simulink model "nonlinear_simulation"  (R2020b)
settings: Solver=ode23t  StartTime=0.0  StopTime=30  MaxStep=0.01  RelTol=1e-7
StopFcn:
  | run plot_simulation_results
values from neighbouring files (symbols this model uses):
  G_hov = [ 0 0 0 0 0 0 1 0 ]    [compute_linear_controller.m]
  G_pos = [ 1 0 0 0 ... (first row only)    [compute_linear_controller.m]
  int_lim = wt/K_hov(5,9) + wt*0.005    [compute_linear_controller.m]
  K_hov = lqr(sys_int, Q, R)    [compute_linear_controller.m]
  K_pos = lqr(sys_hint, Q_pos, R_pos)    [compute_linear_controller.m]
libraries: simulink x1
settings Model: Creator=theso  LastModifiedBy=Emil

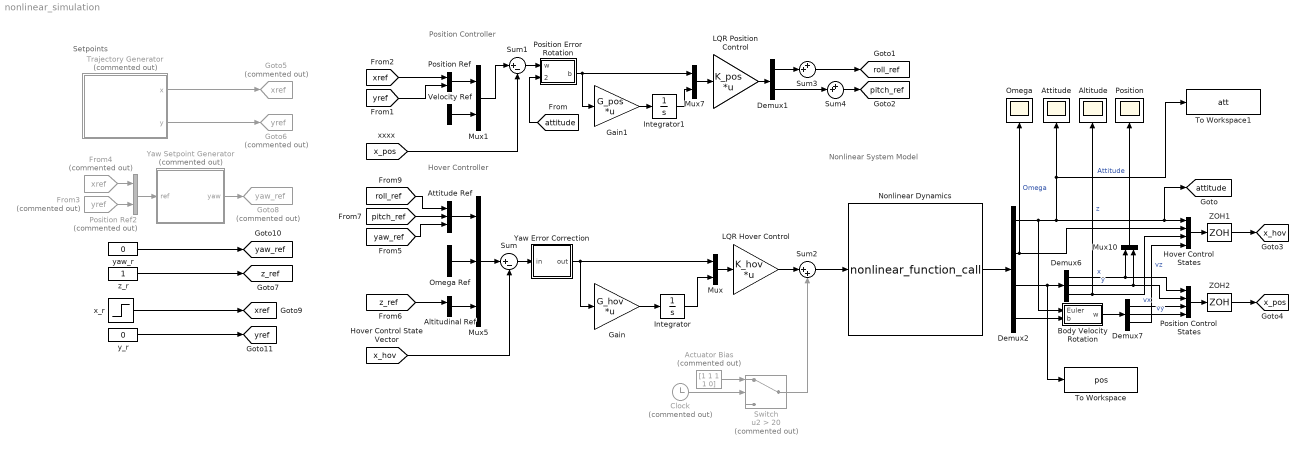
== system nonlinear_simulation ==
  note: Position Controller
  note: Nonlinear System Model
  note: Hover Controller
  note: Setpoints
  Actuator Bias : Constant  Commented=on  Value=[1 1 1 1 0]
  Altitude : Scope
  Altitudinal Ref : Mux  Inputs=2
  Attitude : Scope
  Attitude Ref : Mux  Inputs=3
  Body Velocity Rotation : Subsystem
  Clock : Clock  Commented=on
  Demux1 : Demux  Outputs=2
  Demux2 : Demux
  Demux6 : Demux  Outputs=3
  Demux7 : Demux  Outputs=3
  From3 : From  Commented=on  GotoTag=yref  TagVisibility=global
  From4 : From  Commented=on  GotoTag=xref  TagVisibility=global
  Gain : Gain  Gain=G_hov  Multiplication=Matrix(K*u)
  Gain1 : Gain  Gain=G_pos  Multiplication=Matrix(K*u)
  Goto5 : Goto  Commented=on  GotoTag=xref  TagVisibility=global
  Goto6 : Goto  Commented=on  GotoTag=yref  TagVisibility=global
  Goto8 : Goto  Commented=on  GotoTag=yaw_ref  TagVisibility=global
  Hover Control States : Mux
  Integrator : Integrator  LimitOutput=on  UpperSaturationLimit=int_lim  LowerSaturationLimit=0
  Integrator1 : Integrator  LimitOutput=on  UpperSaturationLimit=0.4  LowerSaturationLimit=-0.4
  LQR Hover Control : Gain  Gain=K_hov  Multiplication=Matrix(K*u)
  LQR Position Control : Gain  Gain=K_pos  Multiplication=Matrix(K*u)
  Mux{,1,7,10} (4 alike) : Mux  Inputs=2
  Mux5 : Mux  Inputs=3
  Nonlinear Dynamics : S-Function  FunctionName=nonlinear_function_call  SFunctionDeploymentMode=off  EnableBusSupport=off
      mask Display: image('drone_model_icon.png'); % Use "Edit Image" on toolstrip to change.
  Omega : Scope
  Omega Ref : Mux  Inputs=3
  Position : Scope
  Position Control States : Mux
  Position Error Rotation : Subsystem
  Position Ref : Mux  Inputs=2
  Position Ref2 : Mux  Commented=on  Inputs=2
  Sum : Sum  Inputs=|+-
  Sum1 : Sum  Inputs=|+-
  Sum2 : Sum  Inputs=|++
  Sum3 : Sum  Inputs=++|
  Sum4 : Sum  Inputs=++|
  Switch : Switch  Commented=on  Criteria=u2 > Threshold  Threshold=20
  To Workspace : ToWorkspace  VariableName=pos  SaveFormat=Timeseries  SampleTime=-1
  To Workspace1 : ToWorkspace  VariableName=att  SaveFormat=Timeseries  SampleTime=-1
  Trajectory Generator : Subsystem  Commented=on
  Velocity Ref : Mux  Inputs=2
  Yaw Error Correction : Subsystem
  Yaw Setpoint Generator : MATLAB Function  Commented=on  TreatAsAtomicUnit=on
  ZOH1 : ZeroOrderHold  SampleTime=0.005
  ZOH2 : ZeroOrderHold  SampleTime=0.005
  x_r : Step  Time=10  SampleTime=0
  y_r : Constant  Value=0
  yaw_r : Constant  Value=0
  z_r : Constant
  tag scope: attitude=global, pitch_ref=global, roll_ref=global, x_hov=global, x_pos=global, xref=global, yaw_ref=global, yref=global, z_ref=global
  wires:
  Mux5/1 -> Sum/1
  Sum/1 -> Yaw Error Correction/1(in)
  Gain/1 -> Integrator/1
  Mux/1 -> LQR Hover Control/1
  Integrator/1 -> Mux/2
  Mux1/1 -> Sum1/1
  Mux7/1 -> LQR Position Control/1
  Nonlinear Dynamics/1 -> Demux2/1
  Demux2/1 -> To Workspace1/1, Attitude/1, [attitude], Hover Control States/1, Body Velocity Rotation/1(Euler)  "Attitude"
  Demux2/2 -> Hover Control States/2, Omega/1  "Omega"
  Demux2/4 -> Body Velocity Rotation/2(b)
  Body Velocity Rotation/1(w) -> Demux7/1
  Demux7/1 -> Position Control States/3  "vx"
  Demux7/2 -> Position Control States/4  "vy"
  Demux6/1 -> Position Control States/1, Mux10/1  "x"
  Demux6/2 -> Mux10/2, Position Control States/2  "y"
  Demux7/3 -> Hover Control States/4  "vz"
  Demux6/3 -> Hover Control States/3, Altitude/1  "z"
  Mux10/1 -> Position/1
  Attitude Ref/1 -> Mux5/1
  Omega Ref/1 -> Mux5/2
  Altitudinal Ref/1 -> Mux5/3
  Velocity Ref/1 -> Mux1/2
  LQR Position Control/1 -> Demux1/1
  Gain1/1 -> Integrator1/1
  Integrator1/1 -> Mux7/2
  Position Ref/1 -> Mux1/1
  Sum1/1 -> Position Error Rotation/1(w)
  Position Error Rotation/1(b) -> Mux7/1, Gain1/1
  Yaw Error Correction/1(out) -> Gain/1, Mux/1
  Demux2/3 -> To Workspace/1, Demux6/1
  [z_ref] -> Altitudinal Ref/1
  [xref] -> Position Ref/1
  [yref] -> Position Ref/2
  [attitude] -> Position Error Rotation/2(Euler)
  From3/1 -> Position Ref2/2
  From4/1 -> Position Ref2/1
  Position Ref2/1 -> Yaw Setpoint Generator/1(ref)
  [yaw_ref] -> Attitude Ref/3
  [roll_ref] -> Attitude Ref/1
  [pitch_ref] -> Attitude Ref/2
  [x_pos] -> Sum1/2
  [x_hov] -> Sum/2
  Hover Control States/1 -> ZOH1/1
  Position Control States/1 -> ZOH2/1
  ZOH1/1 -> [x_hov]
  ZOH2/1 -> [x_pos]
  Trajectory Generator/1(x) -> Goto5/1
  Trajectory Generator/2(y) -> Goto6/1
  z_r/1 -> [z_ref]
  Yaw Setpoint Generator/1(yaw) -> Goto8/1
  x_r/1 -> [xref]
  Clock/1 -> Switch/2
  Actuator Bias/1 -> Switch/1
  LQR Hover Control/1 -> Sum2/1
  Switch/1 -> Sum2/2
  Sum2/1 -> Nonlinear Dynamics/1
  yaw_r/1 -> [yaw_ref]
  y_r/1 -> [yref]
  Demux1/1 -> Sum3/2
  Sum3/1 -> [roll_ref]
  Demux1/2 -> Sum4/2
  Sum4/1 -> [pitch_ref]

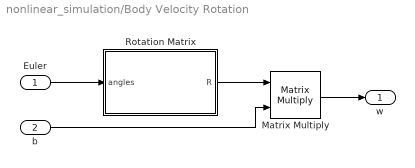
== system nonlinear_simulation/Body Velocity Rotation ==
  Euler : Inport
  b : Inport  Port=2
  Matrix Multiply : Product  Multiplication=Matrix(*)
  Rotation Matrix : MATLAB Function  TreatAsAtomicUnit=on
  w : Outport
  wires:
  Rotation Matrix/1(R) -> Matrix Multiply/1
  Euler/1 -> Rotation Matrix/1(angles)
  b/1 -> Matrix Multiply/2
  Matrix Multiply/1 -> w/1

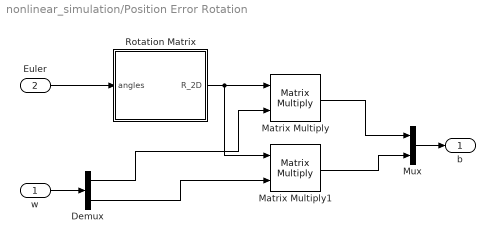
== system nonlinear_simulation/Position Error Rotation ==
  w : Inport
  Euler : Inport  Port=2
  Demux : Demux  Outputs=2
  Matrix Multiply : Product  Multiplication=Matrix(*)
  Matrix Multiply1 : Product  Multiplication=Matrix(*)
  Mux : Mux  Inputs=2
  Rotation Matrix : MATLAB Function  TreatAsAtomicUnit=on
  b : Outport
  wires:
  Rotation Matrix/1(R_2D) -> Matrix Multiply1/1, Matrix Multiply/1
  Euler/1 -> Rotation Matrix/1(angles)
  Matrix Multiply/1 -> Mux/1
  w/1 -> Demux/1
  Demux/2 -> Matrix Multiply1/2
  Demux/1 -> Matrix Multiply/2
  Matrix Multiply1/1 -> Mux/2
  Mux/1 -> b/1

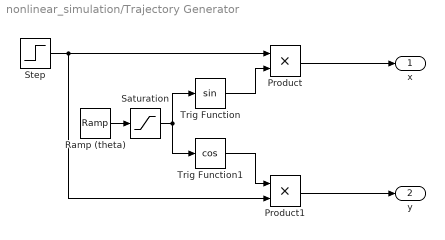
== system nonlinear_simulation/Trajectory Generator ==
  Product : Product  RndMeth=Zero
  Product1 : Product  RndMeth=Zero
  Ramp (theta) : simulink/Sources/Ramp  slope=pi / 20  start=20  InitialOutput=0
  Saturation : Saturate  UpperLimit=2 * pi  LowerLimit=0
  Step : Step  Time=20  SampleTime=0
  Trig Function : Trigonometry
  Trig Function1 : Trigonometry  Operator=cos
  x : Outport
  y : Outport  Port=2
  wires:
  Product/1 -> x/1
  Step/1 -> Product1/2, Product/1
  Ramp (theta)/1 -> Saturation/1
  Trig Function1/1 -> Product1/1
  Saturation/1 -> Trig Function/1, Trig Function1/1
  Trig Function/1 -> Product/2
  Product1/1 -> y/1

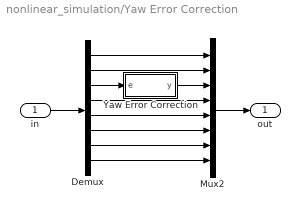
== system nonlinear_simulation/Yaw Error Correction ==
  in : Inport
  Demux : Demux  Outputs=8
  Mux2 : Mux  Inputs=8
  Yaw Error Correction : MATLAB Function  TreatAsAtomicUnit=on
  out : Outport
  wires:
  Demux/8 -> Mux2/8
  Demux/2 -> Mux2/2
  Yaw Error Correction/1(y) -> Mux2/3
  Demux/1 -> Mux2/1
  Demux/3 -> Yaw Error Correction/1(e)
  Demux/7 -> Mux2/7
  Demux/6 -> Mux2/6
  Demux/4 -> Mux2/4
  Demux/5 -> Mux2/5
  Mux2/1 -> out/1
  in/1 -> Demux/1

== matlab function nonlinear_simulation/Yaw Setpoint Generator ==
  settings: updateMethod=DISCRETE
  data: ref input; yaw output size=1
function yaw = yaw_setpoint(ref)

persistent last_ref

if isempty(last_ref)
    last_ref = ref;
end

dx = ref(1) - last_ref(1);
dy = ref(2) - last_ref(2);

last_ref = ref;

yaw = atan2( dy, dx );

== matlab function nonlinear_simulation/Position Error Rotation/Rotation Matrix ==
  data: angles input size=[3 1]; R_2D output size=[2 2]
function R_2D = world_to_body( angles )

    p = 0;
    q = 0;
    u = angles(3);
    
    R_2D = [ cos(q)*cos(u),                         cos(q)*sin(u),                        ;
             cos(u)*sin(p)*sin(q) - cos(p)*sin(u),  cos(p)*cos(u) + sin(p)*sin(q)*sin(u) ];

== matlab function nonlinear_simulation/Yaw Error Correction/Yaw Error Correction ==
  data: e input; y output
function y = fcn(e)
    
    % Correct yaw error
    if( e > pi )
        e = e - 2 * pi;
    end
    
    y = e;
    
end

== matlab function nonlinear_simulation/Body Velocity Rotation/Rotation Matrix ==
  data: angles input size=[3 1]; R output size=[3 3]
function R = body_to_world( angles )

    p = angles(1);
    q = angles(2);
    u = angles(3);
    

    R = [cos(q)*cos(u), sin(p)*sin(q)*cos(u)-cos(p)*sin(u), cos(p)*sin(q)*cos(u)+sin(p)*sin(u) ;
         cos(q)*sin(u), sin(p)*sin(q)*sin(u)+cos(p)*cos(u), cos(p)*sin(q)*sin(u)-sin(p)*cos(u) ;
         -sin(q),       sin(p)*cos(q),                      cos(p)*cos(q)                     ];
